simulink model "LQR_Controller"  (R2018b)
settings: Solver=VariableStepAuto  StartTime=0.0  StopTime=10.0  RelTol=1e-3
undefined symbols (not defined in the file): K, l1, l2, M, m1, m2
settings Model: Creator=Dipam  LastModifiedBy=Dipam

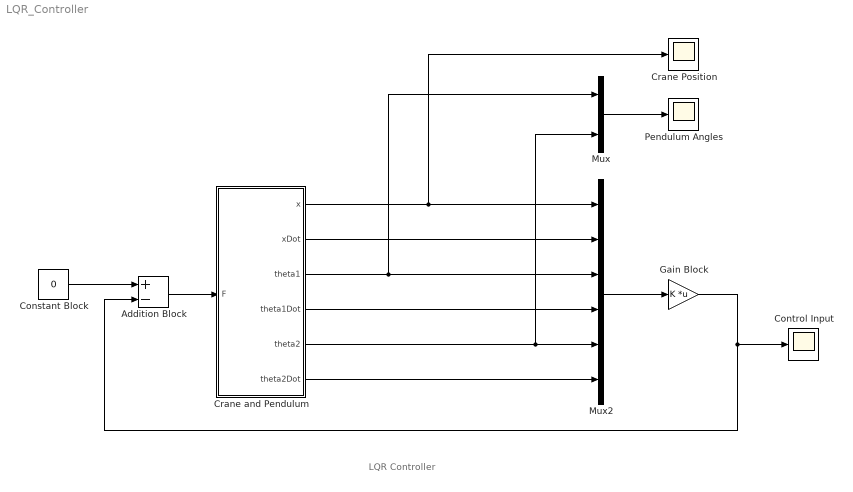
== system LQR_Controller ==
  note: LQR Controller
  Addition Block : Sum  Inputs=+-
  Constant Block : Constant  Value=0
  Control Input : Scope
  Crane Position : Scope
  Crane and Pendulum : Subsystem
  Gain Block : Gain  Gain=K  Multiplication=Matrix(K*u)
  Mux : Mux  Inputs=2
  Mux2 : Mux  Inputs=6
  Pendulum Angles : Scope
  wires:
  Crane and Pendulum/3(theta1) -> Mux/1, Mux2/3
  Crane and Pendulum/4(theta1Dot) -> Mux2/4
  Mux2/1 -> Gain Block/1
  Crane and Pendulum/1(x) -> Mux2/1, Crane Position/1
  Mux/1 -> Pendulum Angles/1
  Crane and Pendulum/5(theta2) -> Mux2/5, Mux/2
  Constant Block/1 -> Addition Block/1
  Crane and Pendulum/2(xDot) -> Mux2/2
  Addition Block/1 -> Crane and Pendulum/1(F)
  Crane and Pendulum/6(theta2Dot) -> Mux2/6
  Gain Block/1 -> Addition Block/2, Control Input/1

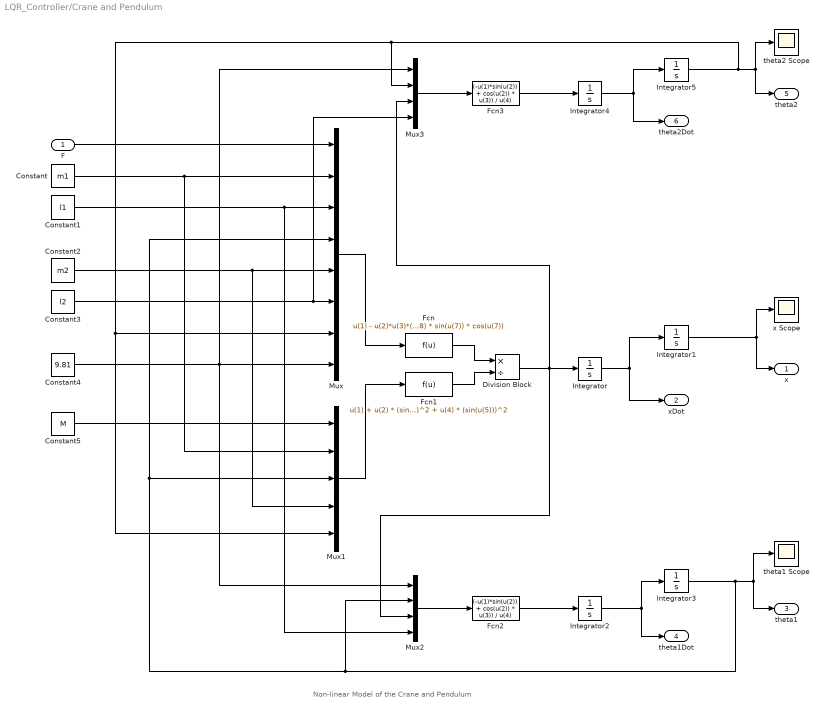
== system LQR_Controller/Crane and Pendulum ==
  note: Non-linear Model of the Crane and Pendulum
  F : Inport
  Constant : Constant  Value=m1
  Constant1 : Constant  Value=l1
  Constant2 : Constant  Value=m2
  Constant3 : Constant  Value=l2
  Constant4 : Constant  Value=9.81
  Constant5 : Constant  Value=M
  Division Block : Product  Inputs=*/
  Fcn : Fcn  Expr=u(1) - u(2)*u(3)*(u(4)^2)*sin(u(4)) - u(5) * u(6) * (u(7)^2)*sin(u(7))-u(2)*u(8)*sin(u(4))*cos(u(4)) - u(5) * u(8) * sin(u(7)) * cos(u(7))
  Fcn1 : Fcn  Expr=u(1) + u(2) * (sin(u(3)))^2 + u(4) * (sin(u(5)))^2
  Fcn2 : Fcn  Expr=(-u(1)*sin(u(2)) + cos(u(2)) * u(3)) / u(4)
  Fcn3 : Fcn  Expr=(-u(1)*sin(u(2)) + cos(u(2)) * u(3)) / u(4)
  Integrator{,1..2,4} (4 alike) : Integrator
  Integrator3 : Integrator  InitialCondition=10*pi/180
  Integrator5 : Integrator  InitialCondition=15*pi/180
  Mux : Mux  Inputs=8
  Mux1 : Mux  Inputs=5
  Mux2 : Mux
  Mux3 : Mux
  theta1 Scope : Scope
  theta2 Scope : Scope
  x Scope : Scope
  x : Outport
  xDot : Outport  Port=2
  theta1 : Outport  Port=3
  theta1Dot : Outport  Port=4
  theta2 : Outport  Port=5
  theta2Dot : Outport  Port=6
  wires:
  Mux1/1 -> Fcn1/1
  Mux3/1 -> Fcn3/1
  Fcn/1 -> Division Block/1
  Integrator2/1 -> Integrator3/1, theta1Dot/1
  Integrator4/1 -> theta2Dot/1, Integrator5/1
  Integrator5/1 -> theta2/1, theta2 Scope/1, Mux1/5, Mux/7, Mux3/2
  Integrator3/1 -> theta1 Scope/1, theta1/1, Mux2/2, Mux/4, Mux1/3
  Division Block/1 -> Mux2/3, Mux3/3, Integrator/1
  Constant5/1 -> Mux1/1
  Constant3/1 -> Mux3/4, Mux/6
  Constant2/1 -> Mux1/4, Mux/5
  Constant/1 -> Mux1/2, Mux/2
  F/1 -> Mux/1
  Constant1/1 -> Mux2/4, Mux/3
  Integrator/1 -> xDot/1, Integrator1/1
  Fcn2/1 -> Integrator2/1
  Constant4/1 -> Mux2/1, Mux/8, Mux3/1
  Mux2/1 -> Fcn2/1
  Integrator1/1 -> x Scope/1, x/1
  Mux/1 -> Fcn/1
  Fcn3/1 -> Integrator4/1
  Fcn1/1 -> Division Block/2
